simulink model "simulink "  (R2022a)
settings: Solver=VariableStepAuto  StartTime=0.0  StopTime=100  RelTol=1e-3
values from neighbouring files (symbols this model uses):
  Lr = Md    [simulink_data .m]
  Lr1 = Md1    [simulink_data .m]
  Lr2 = Md2    [simulink_data .m]
  Mr = Mr-Ld    [simulink_data .m]
  Mr1 = Mr1-Ld1    [simulink_data .m]
  Mr2 = Mr2-Ld2    [simulink_data .m]
  tp = 0.1    [simulink_data .m]
  tp1 = 0.05    [simulink_data .m]
  tp2 = 0.1    [simulink_data .m]
undefined symbols (not defined in the file or in its folder): Ld, Ld1, Ld2, Ld4, Lr4, Md, Md1, Md2, Md4, Mr4
libraries: slpidlib x3
settings Model: Creator=jakubwisniewski  LastModifiedBy=jakubwisniewski

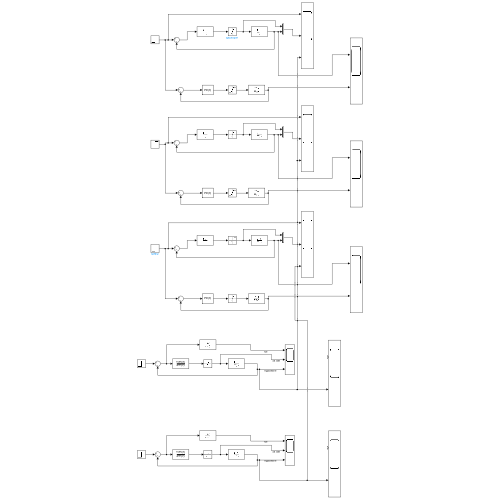
[thumbnail: Simulink's stored preview of the top-level diagram]
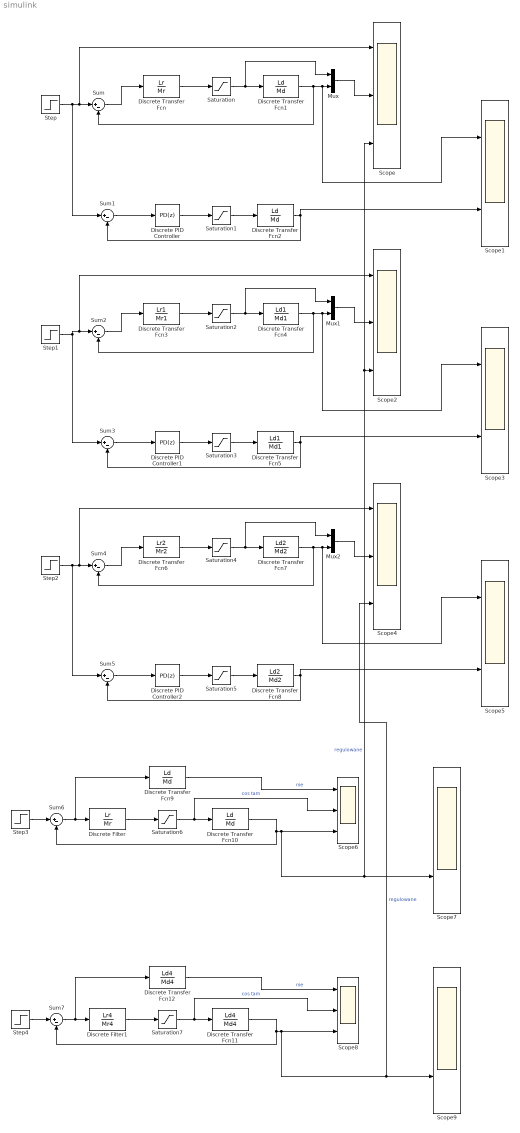
== system simulink  ==
  Discrete Transfer Fcn : DiscreteTransferFcn  Numerator=Lr  Denominator=Mr  SampleTime=tp
  Discrete Transfer Fcn1 : DiscreteTransferFcn  Numerator=Ld  Denominator=Md  SampleTime=tp
  Discrete Transfer Fcn10 : DiscreteTransferFcn  Numerator=Ld  Denominator=Md  SampleTime=0.1
  Discrete Transfer Fcn11 : DiscreteTransferFcn  Numerator=Ld4  Denominator=Md4  SampleTime=0.1
  Discrete Transfer Fcn12 : DiscreteTransferFcn  Numerator=Ld4  Denominator=Md4  SampleTime=0.1
  Discrete Transfer Fcn2 : DiscreteTransferFcn  Numerator=Ld  Denominator=Md
  Discrete Transfer Fcn3 : DiscreteTransferFcn  Numerator=Lr1  Denominator=Mr1  SampleTime=tp1
  Discrete Transfer Fcn4 : DiscreteTransferFcn  Numerator=Ld1  Denominator=Md1  SampleTime=tp1
  Discrete Transfer Fcn5 : DiscreteTransferFcn  Numerator=Ld1  Denominator=Md1  SampleTime=tp1
  Discrete Transfer Fcn6 : DiscreteTransferFcn  Numerator=Lr2  Denominator=Mr2  SampleTime=tp2
  Discrete Transfer Fcn7 : DiscreteTransferFcn  Numerator=Ld2  Denominator=Md2  SampleTime=tp2
  Discrete Transfer Fcn8 : DiscreteTransferFcn  Numerator=Ld2  Denominator=Md2  SampleTime=tp1
  Discrete Transfer Fcn9 : DiscreteTransferFcn  Numerator=Ld  Denominator=Md  SampleTime=0.1
  Discrete Filter : DiscreteFilter  Numerator=Lr  Denominator=Mr  SampleTime=0.1
  Discrete Filter1 : DiscreteFilter  Numerator=Lr4  Denominator=Mr4  SampleTime=0.1
  Discrete PID Controller : slpidlib/PID Controller  Controller=PD  Form=Parallel  TimeDomain=Discrete-time  UseExternalTs=off  SampleTime=tp  IntegratorMethod=Forward Euler  FilterMethod=Forward Euler  ControllerParametersSource=internal  P=0.202306658934468  I=1  UseKiTs=off  D=0.0898307858296902  N=10.5955630231692  UseFilter=on  TunerSelectOption=Transfer Function Based (PID Tuner App)  InitialConditionSource=internal  InitialConditionForIntegrator=0  InitialConditionForFilter=0  DifferentiatorICPrevScaledInput=0  ExternalReset=none  TrackingMode=off  Kt=1  LimitOutput=off  SatLimitsSource=internal  UpperSaturationLimit=inf  LowerSaturationLimit=-inf  LinearizeAsGain=off  AntiWindupMode=none  Kb=1  POutMin=[]  POutMax=[]  IOutMin=[]  IOutMax=[]  DOutMin=[]  DOutMax=[]  NOutMin=[]  NOutMax=[]  SumOutMin=[]  SumOutMax=[]  SaturationOutMin=[]  SaturationOutMax=[]  PParamMin=[]  PParamMax=[]  IParamMin=[]  IParamMax=[]  DParamMin=[]  DParamMax=[]  NParamMin=[]  NParamMax=[]  KbParamMin=[]  KbParamMax=[]  KtParamMin=[]  KtParamMax=[]  KbOutMin=[]  KbOutMax=[]  KtOutMin=[]  KtOutMax=[]  IntegratorOutMin=[]  IntegratorOutMax=[]  FilterOutMin=[]  FilterOutMax=[]  SumI1OutMin=[]  SumI1OutMax=[]  SumI2OutMin=[]  SumI2OutMax=[]  SumI3OutMin=[]  SumI3OutMax=[]  SumI4OutMin=[]  SumI4OutMax=[]  SumDOutMin=[]  SumDOutMax=[]  DifferentiatorOutMin=[]  DifferentiatorOutMax=[]  FilterDiffOutCoefMin=[]  FilterDiffOutCoefMax=[]  ReciprocalOutMin=[]  ReciprocalOutMax=[]  SumDenOutMin=[]  SumDenOutMax=[]  SumNumOutMin=[]  SumNumOutMax=[]  DivideOutMin=[]  DivideOutMax=[]  UdiffTsProdOutMin=[]  UdiffTsProdOutMax=[]  NTsProdOutMin=[]  NTsProdOutMax=[]  UintegralTsProdOutMin=[]  UintegralTsProdOutMax=[]  UngainTsProdOutMin=[]  UngainTsProdOutMax=[]  IntegratorContinuousStateAttributes=''  IntegratorStateMustResolveToSignalObject=off  IntegratorRTWStateStorageClass=Auto  FilterContinuousStateAttributes=''  FilterStateMustResolveToSignalObject=off  FilterRTWStateStorageClass=Auto  ParallelPVariant=InternalParameters  IdealPVariant=Disabled  IVariant=Disabled  DVariant=InternalParameters  IntegratorVariant=Disabled  SatVariant=Disabled  AWVariant=Disabled  PCopyVariant=Disabled  TRVariant=Disabled  FdbkBlocksVariant=Forward  IdealPFdbkVariant=Disabled  SatFdbkVariant=Disabled  DerivativeFilterVariant=ForwardEulerFilter  NVariant=InternalParameters  NCopyVariant=Disabled  FilterICVariant=InternalICsFilter  IntegratorICVariant=Disabled  ExternalResetVariant=Disabled  TRSumVariant=Passthrough  SumFdbkVariant=Disabled  SumVariant=Sum_PD  TsampFilterVariant=InternalTs  TsampNgainVariant=Passthrough  TsampIntegralVariant=Disabled_SignalSpec  ExternalSaturationOutDataTypeStr=Inherit: Same as second input  aMode=0
  Discrete PID Controller1 : slpidlib/PID Controller  Controller=PD  Form=Parallel  TimeDomain=Discrete-time  UseExternalTs=off  SampleTime=tp  IntegratorMethod=Forward Euler  FilterMethod=Forward Euler  ControllerParametersSource=internal  P=0.202306658934468  I=1  UseKiTs=off  D=0.0898307858296902  N=10.5955630231692  UseFilter=on  TunerSelectOption=Transfer Function Based (PID Tuner App)  InitialConditionSource=internal  InitialConditionForIntegrator=0  InitialConditionForFilter=0  DifferentiatorICPrevScaledInput=0  ExternalReset=none  TrackingMode=off  Kt=1  LimitOutput=off  SatLimitsSource=internal  UpperSaturationLimit=inf  LowerSaturationLimit=-inf  LinearizeAsGain=off  AntiWindupMode=none  Kb=1  POutMin=[]  POutMax=[]  IOutMin=[]  IOutMax=[]  DOutMin=[]  DOutMax=[]  NOutMin=[]  NOutMax=[]  SumOutMin=[]  SumOutMax=[]  SaturationOutMin=[]  SaturationOutMax=[]  PParamMin=[]  PParamMax=[]  IParamMin=[]  IParamMax=[]  DParamMin=[]  DParamMax=[]  NParamMin=[]  NParamMax=[]  KbParamMin=[]  KbParamMax=[]  KtParamMin=[]  KtParamMax=[]  KbOutMin=[]  KbOutMax=[]  KtOutMin=[]  KtOutMax=[]  IntegratorOutMin=[]  IntegratorOutMax=[]  FilterOutMin=[]  FilterOutMax=[]  SumI1OutMin=[]  SumI1OutMax=[]  SumI2OutMin=[]  SumI2OutMax=[]  SumI3OutMin=[]  SumI3OutMax=[]  SumI4OutMin=[]  SumI4OutMax=[]  SumDOutMin=[]  SumDOutMax=[]  DifferentiatorOutMin=[]  DifferentiatorOutMax=[]  FilterDiffOutCoefMin=[]  FilterDiffOutCoefMax=[]  ReciprocalOutMin=[]  ReciprocalOutMax=[]  SumDenOutMin=[]  SumDenOutMax=[]  SumNumOutMin=[]  SumNumOutMax=[]  DivideOutMin=[]  DivideOutMax=[]  UdiffTsProdOutMin=[]  UdiffTsProdOutMax=[]  NTsProdOutMin=[]  NTsProdOutMax=[]  UintegralTsProdOutMin=[]  UintegralTsProdOutMax=[]  UngainTsProdOutMin=[]  UngainTsProdOutMax=[]  IntegratorContinuousStateAttributes=''  IntegratorStateMustResolveToSignalObject=off  IntegratorRTWStateStorageClass=Auto  FilterContinuousStateAttributes=''  FilterStateMustResolveToSignalObject=off  FilterRTWStateStorageClass=Auto  ParallelPVariant=InternalParameters  IdealPVariant=Disabled  IVariant=Disabled  DVariant=InternalParameters  IntegratorVariant=Disabled  SatVariant=Disabled  AWVariant=Disabled  PCopyVariant=Disabled  TRVariant=Disabled  FdbkBlocksVariant=Forward  IdealPFdbkVariant=Disabled  SatFdbkVariant=Disabled  DerivativeFilterVariant=ForwardEulerFilter  NVariant=InternalParameters  NCopyVariant=Disabled  FilterICVariant=InternalICsFilter  IntegratorICVariant=Disabled  ExternalResetVariant=Disabled  TRSumVariant=Passthrough  SumFdbkVariant=Disabled  SumVariant=Sum_PD  TsampFilterVariant=InternalTs  TsampNgainVariant=Passthrough  TsampIntegralVariant=Disabled_SignalSpec  ExternalSaturationOutDataTypeStr=Inherit: Same as second input  aMode=0
  Discrete PID Controller2 : slpidlib/PID Controller  Controller=PD  Form=Parallel  TimeDomain=Discrete-time  UseExternalTs=off  SampleTime=tp2  IntegratorMethod=Forward Euler  FilterMethod=Forward Euler  ControllerParametersSource=internal  P=0.202306658934468  I=1  UseKiTs=off  D=0.0898307858296902  N=10.5955630231692  UseFilter=on  TunerSelectOption=Transfer Function Based (PID Tuner App)  InitialConditionSource=internal  InitialConditionForIntegrator=0  InitialConditionForFilter=0  DifferentiatorICPrevScaledInput=0  ExternalReset=none  TrackingMode=off  Kt=1  LimitOutput=off  SatLimitsSource=internal  UpperSaturationLimit=inf  LowerSaturationLimit=-inf  LinearizeAsGain=off  AntiWindupMode=none  Kb=1  POutMin=[]  POutMax=[]  IOutMin=[]  IOutMax=[]  DOutMin=[]  DOutMax=[]  NOutMin=[]  NOutMax=[]  SumOutMin=[]  SumOutMax=[]  SaturationOutMin=[]  SaturationOutMax=[]  PParamMin=[]  PParamMax=[]  IParamMin=[]  IParamMax=[]  DParamMin=[]  DParamMax=[]  NParamMin=[]  NParamMax=[]  KbParamMin=[]  KbParamMax=[]  KtParamMin=[]  KtParamMax=[]  KbOutMin=[]  KbOutMax=[]  KtOutMin=[]  KtOutMax=[]  IntegratorOutMin=[]  IntegratorOutMax=[]  FilterOutMin=[]  FilterOutMax=[]  SumI1OutMin=[]  SumI1OutMax=[]  SumI2OutMin=[]  SumI2OutMax=[]  SumI3OutMin=[]  SumI3OutMax=[]  SumI4OutMin=[]  SumI4OutMax=[]  SumDOutMin=[]  SumDOutMax=[]  DifferentiatorOutMin=[]  DifferentiatorOutMax=[]  FilterDiffOutCoefMin=[]  FilterDiffOutCoefMax=[]  ReciprocalOutMin=[]  ReciprocalOutMax=[]  SumDenOutMin=[]  SumDenOutMax=[]  SumNumOutMin=[]  SumNumOutMax=[]  DivideOutMin=[]  DivideOutMax=[]  UdiffTsProdOutMin=[]  UdiffTsProdOutMax=[]  NTsProdOutMin=[]  NTsProdOutMax=[]  UintegralTsProdOutMin=[]  UintegralTsProdOutMax=[]  UngainTsProdOutMin=[]  UngainTsProdOutMax=[]  IntegratorContinuousStateAttributes=''  IntegratorStateMustResolveToSignalObject=off  IntegratorRTWStateStorageClass=Auto  FilterContinuousStateAttributes=''  FilterStateMustResolveToSignalObject=off  FilterRTWStateStorageClass=Auto  ParallelPVariant=InternalParameters  IdealPVariant=Disabled  IVariant=Disabled  DVariant=InternalParameters  IntegratorVariant=Disabled  SatVariant=Disabled  AWVariant=Disabled  PCopyVariant=Disabled  TRVariant=Disabled  FdbkBlocksVariant=Forward  IdealPFdbkVariant=Disabled  SatFdbkVariant=Disabled  DerivativeFilterVariant=ForwardEulerFilter  NVariant=InternalParameters  NCopyVariant=Disabled  FilterICVariant=InternalICsFilter  IntegratorICVariant=Disabled  ExternalResetVariant=Disabled  TRSumVariant=Passthrough  SumFdbkVariant=Disabled  SumVariant=Sum_PD  TsampFilterVariant=InternalTs  TsampNgainVariant=Passthrough  TsampIntegralVariant=Disabled_SignalSpec  ExternalSaturationOutDataTypeStr=Inherit: Same as second input  aMode=0
  Mux : Mux  Inputs=2
  Mux1 : Mux  Inputs=2
  Mux2 : Mux  Inputs=2
  Saturation{,2,4,6..7} (5 alike) : Saturate  UpperLimit=100  LowerLimit=-100
  Saturation1 : Saturate  UpperLimit=1  LowerLimit=-1
  Saturation3 : Saturate  UpperLimit=1  LowerLimit=-1
  Saturation5 : Saturate  UpperLimit=1  LowerLimit=-1
  Scope{,2,4,6,8} (5 alike) : Scope  NumInputPorts=3
  Scope{1,3,5,7,9} (5 alike) : Scope  NumInputPorts=2
  Step : Step  SampleTime=tp
  Step1 : Step  SampleTime=tp1
  Step2 : Step  SampleTime=tp2
  Step3 : Step  SampleTime=0.1
  Step4 : Step  SampleTime=0.1
  Sum{,1..7} (8 alike) : Sum  Inputs=|+-
  wires:
  Discrete Transfer Fcn/1 -> Saturation/1
  Saturation/1 -> Discrete Transfer Fcn1/1, Mux/1
  Step/1 -> Sum1/1, Scope/1, Sum/1
  Sum/1 -> Discrete Transfer Fcn/1
  Discrete Transfer Fcn1/1 -> Scope1/1, Mux/2, Sum/2
  Discrete PID Controller/1 -> Saturation1/1
  Saturation1/1 -> Discrete Transfer Fcn2/1
  Sum1/1 -> Discrete PID Controller/1
  Mux/1 -> Scope/2
  Discrete Transfer Fcn2/1 -> Scope1/2, Sum1/2
  Mux1/1 -> Scope2/2
  Saturation2/1 -> Discrete Transfer Fcn4/1, Mux1/1
  Discrete Transfer Fcn5/1 -> Scope3/2, Sum3/2
  Sum2/1 -> Discrete Transfer Fcn3/1
  Sum3/1 -> Discrete PID Controller1/1
  Saturation3/1 -> Discrete Transfer Fcn5/1
  Discrete Transfer Fcn4/1 -> Scope3/1, Mux1/2, Sum2/2
  Discrete PID Controller1/1 -> Saturation3/1
  Discrete Transfer Fcn3/1 -> Saturation2/1
  Step1/1 -> Scope2/1, Sum2/1, Sum3/1
  Saturation4/1 -> Discrete Transfer Fcn7/1, Mux2/1
  Discrete Transfer Fcn8/1 -> Scope5/2, Sum5/2
  Discrete PID Controller2/1 -> Saturation5/1
  Mux2/1 -> Scope4/2
  Sum5/1 -> Discrete PID Controller2/1
  Discrete Transfer Fcn7/1 -> Scope5/1, Mux2/2, Sum4/2
  Saturation5/1 -> Discrete Transfer Fcn8/1
  Sum4/1 -> Discrete Transfer Fcn6/1
  Discrete Transfer Fcn6/1 -> Saturation4/1
  Step2/1 -> Sum5/1, Scope4/1, Sum4/1
  Discrete Filter/1 -> Saturation6/1
  Saturation6/1 -> Discrete Transfer Fcn10/1, Scope6/2  "cos tam"
  Discrete Transfer Fcn10/1 -> Scope7/2, Scope/3, Scope2/3, Scope6/3, Sum6/2  "regulowane"
  Sum6/1 -> Discrete Transfer Fcn9/1, Discrete Filter/1
  Discrete Transfer Fcn9/1 -> Scope6/1  "nie"
  Step3/1 -> Sum6/1
  Discrete Transfer Fcn11/1 -> Scope4/3, Scope9/2, Scope8/3, Sum7/2  "regulowane"
  Discrete Filter1/1 -> Saturation7/1
  Sum7/1 -> Discrete Transfer Fcn12/1, Discrete Filter1/1
  Saturation7/1 -> Discrete Transfer Fcn11/1, Scope8/2  "cos tam"
  Discrete Transfer Fcn12/1 -> Scope8/1  "nie"
  Step4/1 -> Sum7/1
